simulink library "libMdl_AccIntegrator"  (R2019b)
settings: Solver=VariableStepAuto  StartTime=0.0  StopTime=10.0  RelTol=1e-3
undefined symbols (not defined in the file): DiscIntNeverNeededParam
libraries: libMdl_crossProdMat x1, libMdl_transformVect x1
settings Model: Creator=Hanno  LastModifiedBy=Hanno

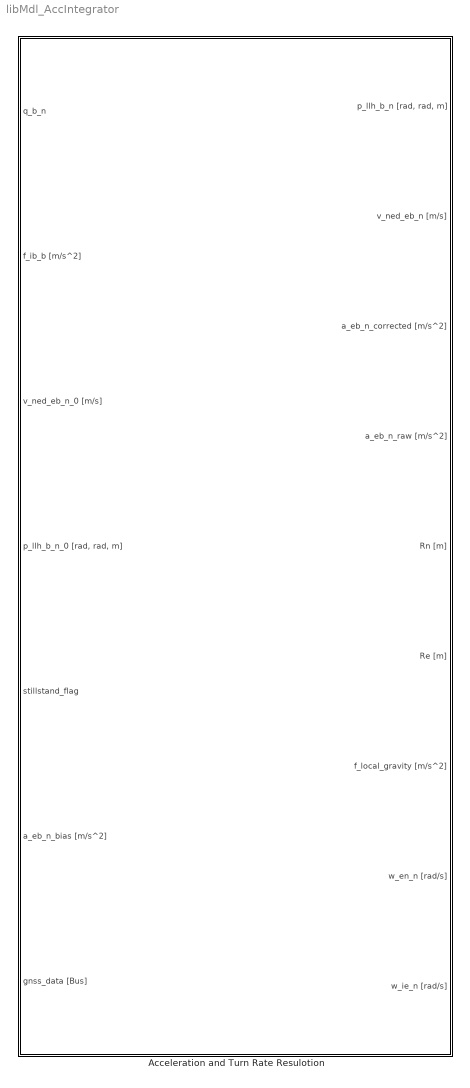
== system libMdl_AccIntegrator ==
  "Acceleration and Turn Rate Resulotion " : Subsystem  mask{mv_sample_time=-1}
      mask prompts: mv_sample_time "Sample Time:"
      mask Display:
      | str1 = sprintf('\\color{black}{\\bfINS Resolution and Integration}\n\n');
      | str2 = sprintf('Sample Time: %0.3f',mv_sample_time);
      | 
      | str = [str1,str2];
      | 
      | text( 0.5,0.5, ...
      |       str, ...
      |       'horizontalAlignment', 'center', ...
      |       'texmode','on' ...
      |     )

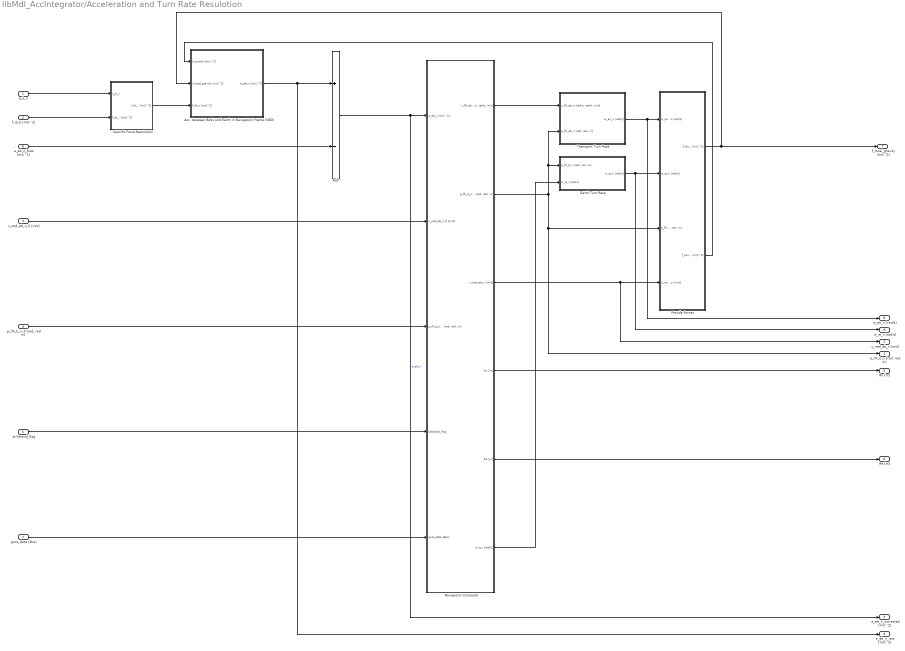
== system libMdl_AccIntegrator/Acceleration and Turn Rate Resulotion  ==
  q_b_n : Inport
  f_ib_b [m/s^2] : Inport  Port=2
  v_ned_eb_n_0 [m/s] : Inport  Port=3
  "p_llh_b_n_0 [rad, rad, m] " : Inport  Port=4
  stillstand_flag : Inport  Port=5
  a_eb_n_bias [m/s^2] : Inport  Port=6
  gnss_data [Bus] : Inport  Port=7
  Acc. between Body and Earth in Navigation Frame (NED) : Subsystem
  Add : Sum  Inputs=+-
  Earth Turn Rate : Subsystem
  Navigation Computer : Subsystem
  Pseude Forces : Subsystem
  Specific Force Resolution : Subsystem
  Transport Turn Rate : Subsystem
  "p_llh_b_n [rad, rad, m]" : Outport  VectorParamsAs1DForOutWhenUnconnected=off
  v_ned_eb_n [m/s] : Outport  Port=2  VectorParamsAs1DForOutWhenUnconnected=off
  a_eb_n_corrected [m/s^2] : Outport  Port=3  VectorParamsAs1DForOutWhenUnconnected=off
  a_eb_n_raw [m/s^2] : Outport  Port=4  VectorParamsAs1DForOutWhenUnconnected=off
  Rn [m] : Outport  Port=5  VectorParamsAs1DForOutWhenUnconnected=off
  Re [m] : Outport  Port=6  VectorParamsAs1DForOutWhenUnconnected=off
  f_local_gravity [m/s^2] : Outport  Port=7  VectorParamsAs1DForOutWhenUnconnected=off
  w_en_n [rad/s] : Outport  Port=8  VectorParamsAs1DForOutWhenUnconnected=off
  w_ie_n [rad/s] : Outport  Port=9  VectorParamsAs1DForOutWhenUnconnected=off
  wires:
  Navigation Computer/6(w_ie_i [rad/s]) -> Earth Turn Rate/2(w_ie_i [rad/s])
  a_eb_n_bias [m/s^2]/1 -> Add/2
  stillstand_flag/1 -> Navigation Computer/4(stillstand_flag)
  Add/1 -> a_eb_n_corrected [m/s^2]/1, Navigation Computer/1(a_eb_n [m/s^2])  "a_eb_n"
  Navigation Computer/5(Re [m]) -> Re [m]/1
  Navigation Computer/4(Rn [m]) -> Rn [m]/1
  Pseude Forces/1(f_local_gravity [m/s^2]) -> Acc. between Body and Earth in Navigation Frame (NED)/2(f_local_gravity [m/s^2]), f_local_gravity [m/s^2]/1
  Pseude Forces/2(f_coriolis [m/s^2]) -> Acc. between Body and Earth in Navigation Frame (NED)/1(f_coriolis [m/s^2])
  Navigation Computer/3(v_ned_eb_n [m/s]) -> Pseude Forces/4(v_ned_eb_n [m/s]), v_ned_eb_n [m/s]/1
  Earth Turn Rate/1(w_ie_n [rad/s]) -> Pseude Forces/2(w_ie_n [rad/s]), w_ie_n [rad/s]/1
  Transport Turn Rate/1(w_en_n [rad/s]) -> w_en_n [rad/s]/1, Pseude Forces/1(w_en_n [rad/s])
  Navigation Computer/1("v_llh_eb_n [rad/s, rad/s, m/s]") -> Transport Turn Rate/1("v_llh_eb_n [rad/s, rad/s, m/s]")
  Navigation Computer/2("p_llh_b_n [rad, rad, m]") -> Earth Turn Rate/1("p_llh_b_n [rad, rad, m]"), Transport Turn Rate/2("p_llh_eb_n [rad, rad, m]"), Pseude Forces/3("p_llh_eb_n [rad, rad, m]"), "p_llh_b_n [rad, rad, m]"/1
  f_ib_b [m/s^2]/1 -> Specific Force Resolution/2(f_ib_b [m/s^2])
  Specific Force Resolution/1(f_ib_n [m/s^2]) -> Acc. between Body and Earth in Navigation Frame (NED)/3(f_ib_n [m/s^2])
  "p_llh_b_n_0 [rad, rad, m] "/1 -> Navigation Computer/3("p_llh_b_n_0 [rad, rad, m]")
  Acc. between Body and Earth in Navigation Frame (NED)/1(a_eb_n [m/s^2]) -> Add/1, a_eb_n_raw [m/s^2]/1
  v_ned_eb_n_0 [m/s]/1 -> Navigation Computer/2(v_ned_eb_n_0 [m/s])
  q_b_n/1 -> Specific Force Resolution/1(q_b_n)
  gnss_data [Bus]/1 -> Navigation Computer/5(gnss_data [Bus])

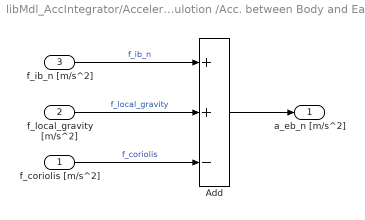
== system libMdl_AccIntegrator/Acceleration and Turn Rate Resulotion /Acc. between Body and Earth in Navigation Frame (NED) ==
  f_coriolis [m/s^2] : Inport
  f_local_gravity [m/s^2] : Inport  Port=2
  f_ib_n [m/s^2] : Inport  Port=3
  Add : Sum  Inputs=++-
  a_eb_n [m/s^2] : Outport  VectorParamsAs1DForOutWhenUnconnected=off
  wires:
  f_coriolis [m/s^2]/1 -> Add/3  "f_coriolis"
  f_local_gravity [m/s^2]/1 -> Add/2  "f_local_gravity"
  Add/1 -> a_eb_n [m/s^2]/1
  f_ib_n [m/s^2]/1 -> Add/1  "f_ib_n"

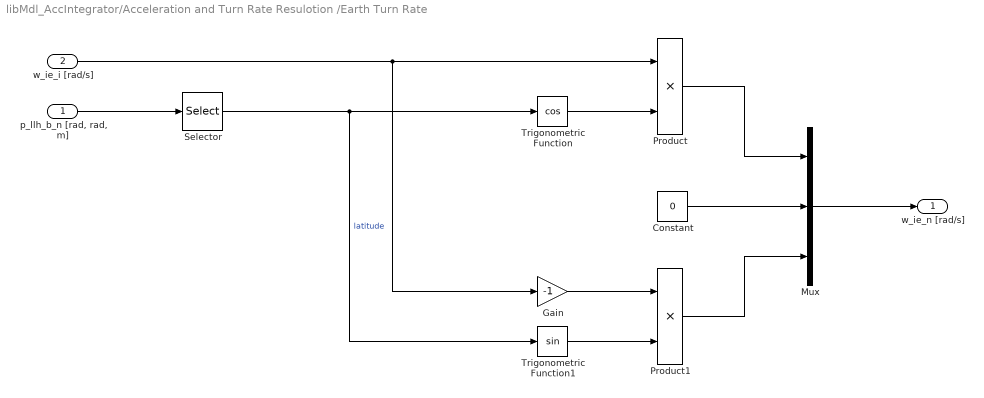
== system libMdl_AccIntegrator/Acceleration and Turn Rate Resulotion /Earth Turn Rate ==
  "p_llh_b_n [rad, rad, m]" : Inport
  w_ie_i [rad/s] : Inport  Port=2
  Constant : Constant  Value=0
  Gain : Gain  Gain=-1
  Mux : Mux  Inputs=3
  Product : Product
  Product1 : Product
  Selector : Selector  InputPortWidth=3  IndexOptions=Index vector (dialog)  Indices=1  OutputSizes=1
  Trigonometric Function : Trigonometry  Operator=cos
  Trigonometric Function1 : Trigonometry
  w_ie_n [rad/s] : Outport  VectorParamsAs1DForOutWhenUnconnected=off
  wires:
  Product1/1 -> Mux/3
  Product/1 -> Mux/1
  Constant/1 -> Mux/2
  Gain/1 -> Product1/1
  Mux/1 -> w_ie_n [rad/s]/1
  Trigonometric Function1/1 -> Product1/2
  Trigonometric Function/1 -> Product/2
  w_ie_i [rad/s]/1 -> Product/1, Gain/1
  Selector/1 -> Trigonometric Function/1, Trigonometric Function1/1  "latitude"
  "p_llh_b_n [rad, rad, m]"/1 -> Selector/1

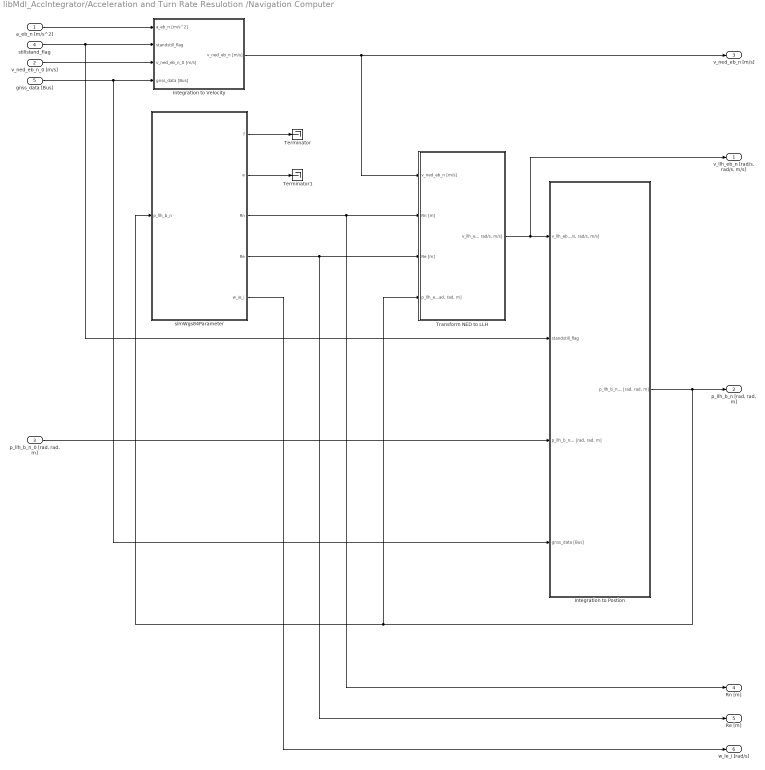
== system libMdl_AccIntegrator/Acceleration and Turn Rate Resulotion /Navigation Computer ==
  a_eb_n [m/s^2] : Inport
  v_ned_eb_n_0 [m/s] : Inport  Port=2
  "p_llh_b_n_0 [rad, rad, m]" : Inport  Port=3
  stillstand_flag : Inport  Port=4
  gnss_data [Bus] : Inport  Port=5
  Integration to Postion : Subsystem
  Integration to Velocity : Subsystem
  Terminator : Terminator
  Terminator1 : Terminator
  Transform NED to LLH : Subsystem
  simWgs84Parameter : MATLAB Function  TreatAsAtomicUnit=on  SystemSampleTime=mv_sample_time  mask{mv_sample_time=-1}
      mask prompts: mv_sample_time "Sample Time:"
  "v_llh_eb_n [rad/s, rad/s, m/s]" : Outport  VectorParamsAs1DForOutWhenUnconnected=off
  "p_llh_b_n [rad, rad, m]" : Outport  Port=2  VectorParamsAs1DForOutWhenUnconnected=off
  v_ned_eb_n [m/s] : Outport  Port=3  VectorParamsAs1DForOutWhenUnconnected=off
  Rn [m] : Outport  Port=4  VectorParamsAs1DForOutWhenUnconnected=off
  Re [m] : Outport  Port=5  VectorParamsAs1DForOutWhenUnconnected=off
  w_ie_i [rad/s] : Outport  Port=6  VectorParamsAs1DForOutWhenUnconnected=off
  wires:
  simWgs84Parameter/5(w_ie_i) -> w_ie_i [rad/s]/1
  stillstand_flag/1 -> Integration to Postion/2(standstill_flag), Integration to Velocity/2(standstill_flag)
  simWgs84Parameter/2(e) -> Terminator1/1
  simWgs84Parameter/1(f) -> Terminator/1
  simWgs84Parameter/4(Re) -> Transform NED to LLH/3(Re [m]), Re [m]/1
  simWgs84Parameter/3(Rn) -> Transform NED to LLH/2(Rn [m]), Rn [m]/1
  Integration to Postion/1("p_llh_b_n [rad, rad, m]") -> "p_llh_b_n [rad, rad, m]"/1, Transform NED to LLH/4("p_llh_eb_n [rad, rad, m]"), simWgs84Parameter/1(p_llh_b_n)
  "p_llh_b_n_0 [rad, rad, m]"/1 -> Integration to Postion/3("p_llh_b_n_0 [rad, rad, m]")
  v_ned_eb_n_0 [m/s]/1 -> Integration to Velocity/3(v_ned_eb_n_0 [m/s])
  Integration to Velocity/1(v_ned_eb_n [m/s]) -> Transform NED to LLH/1(v_ned_eb_n [m/s]), v_ned_eb_n [m/s]/1
  a_eb_n [m/s^2]/1 -> Integration to Velocity/1(a_eb_n [m/s^2])
  Transform NED to LLH/1("v_llh_eb_n [rad/s, rad/s, m/s]") -> "v_llh_eb_n [rad/s, rad/s, m/s]"/1, Integration to Postion/1("v_llh_eb_n [rad/s, rad/s, m/s]")
  gnss_data [Bus]/1 -> Integration to Velocity/4(gnss_data [Bus]), Integration to Postion/4(gnss_data [Bus])

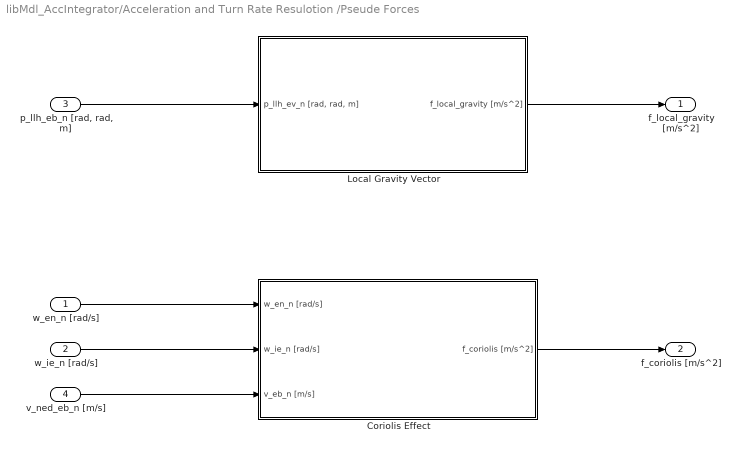
== system libMdl_AccIntegrator/Acceleration and Turn Rate Resulotion /Pseude Forces ==
  w_en_n [rad/s] : Inport
  w_ie_n [rad/s] : Inport  Port=2
  "p_llh_eb_n [rad, rad, m]" : Inport  Port=3
  v_ned_eb_n [m/s] : Inport  Port=4
  Coriolis Effect : Subsystem
  Local Gravity Vector : Subsystem
      settings: AttributesFormatString="Local Gravity Model according to: D. Titterton and J. Westen, \"Strapdown Inertial Navigation Technology\", p. 57, IET, 2004"
  f_local_gravity [m/s^2] : Outport  VectorParamsAs1DForOutWhenUnconnected=off
  f_coriolis [m/s^2] : Outport  Port=2  VectorParamsAs1DForOutWhenUnconnected=off
  wires:
  Coriolis Effect/1(f_coriolis [m/s^2]) -> f_coriolis [m/s^2]/1
  Local Gravity Vector/1(f_local_gravity [m/s^2]) -> f_local_gravity [m/s^2]/1
  v_ned_eb_n [m/s]/1 -> Coriolis Effect/3(v_eb_n [m/s])
  "p_llh_eb_n [rad, rad, m]"/1 -> Local Gravity Vector/1("p_llh_ev_n [rad, rad, m]")
  w_ie_n [rad/s]/1 -> Coriolis Effect/2(w_ie_n [rad/s])
  w_en_n [rad/s]/1 -> Coriolis Effect/1(w_en_n [rad/s])

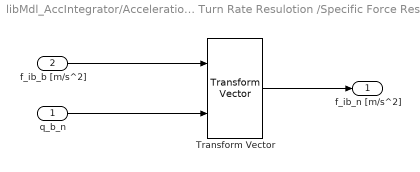
== system libMdl_AccIntegrator/Acceleration and Turn Rate Resulotion /Specific Force Resolution ==
  q_b_n : Inport
  f_ib_b [m/s^2] : Inport  Port=2
  Transform Vector : libMdl_transformVect/Transform Vector  SystemSampleTime=-1  Latency=0  AutoFrameSizeCalculation=off
  f_ib_n [m/s^2] : Outport  VectorParamsAs1DForOutWhenUnconnected=off
  wires:
  f_ib_b [m/s^2]/1 -> Transform Vector/1
  Transform Vector/1 -> f_ib_n [m/s^2]/1
  q_b_n/1 -> Transform Vector/2

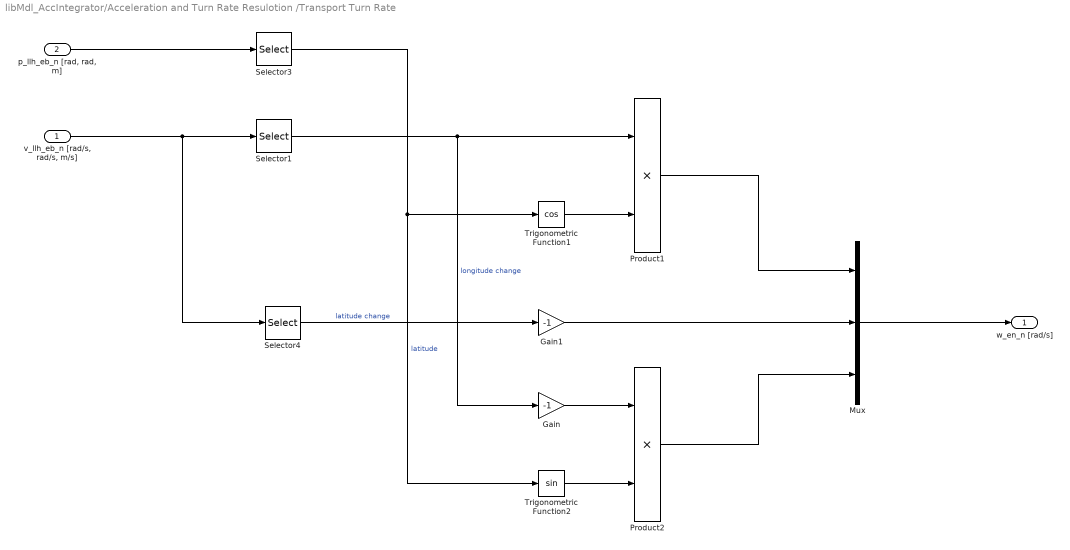
== system libMdl_AccIntegrator/Acceleration and Turn Rate Resulotion /Transport Turn Rate ==
  "v_llh_eb_n [rad/s, rad/s, m/s]" : Inport
  "p_llh_eb_n [rad, rad, m]" : Inport  Port=2
  Gain : Gain  Gain=-1
  Gain1 : Gain  Gain=-1
  Mux : Mux  Inputs=3
  Product1 : Product
  Product2 : Product
  Selector1 : Selector  InputPortWidth=3  IndexOptions=Index vector (dialog)  Indices=2  OutputSizes=1
  Selector3 : Selector  InputPortWidth=3  IndexOptions=Index vector (dialog)  Indices=1  OutputSizes=1
  Selector4 : Selector  InputPortWidth=3  IndexOptions=Index vector (dialog)  Indices=1  OutputSizes=1
  Trigonometric Function1 : Trigonometry  Operator=cos
  Trigonometric Function2 : Trigonometry
  w_en_n [rad/s] : Outport  VectorParamsAs1DForOutWhenUnconnected=off
  wires:
  Product2/1 -> Mux/3
  Product1/1 -> Mux/1
  Gain1/1 -> Mux/2
  Gain/1 -> Product2/1
  Trigonometric Function2/1 -> Product2/2
  Selector4/1 -> Gain1/1  "latitude change"
  Selector1/1 -> Product1/1, Gain/1  "longitude change"
  Selector3/1 -> Trigonometric Function1/1, Trigonometric Function2/1  "latitude"
  Trigonometric Function1/1 -> Product1/2
  Mux/1 -> w_en_n [rad/s]/1
  "p_llh_eb_n [rad, rad, m]"/1 -> Selector3/1
  "v_llh_eb_n [rad/s, rad/s, m/s]"/1 -> Selector1/1, Selector4/1

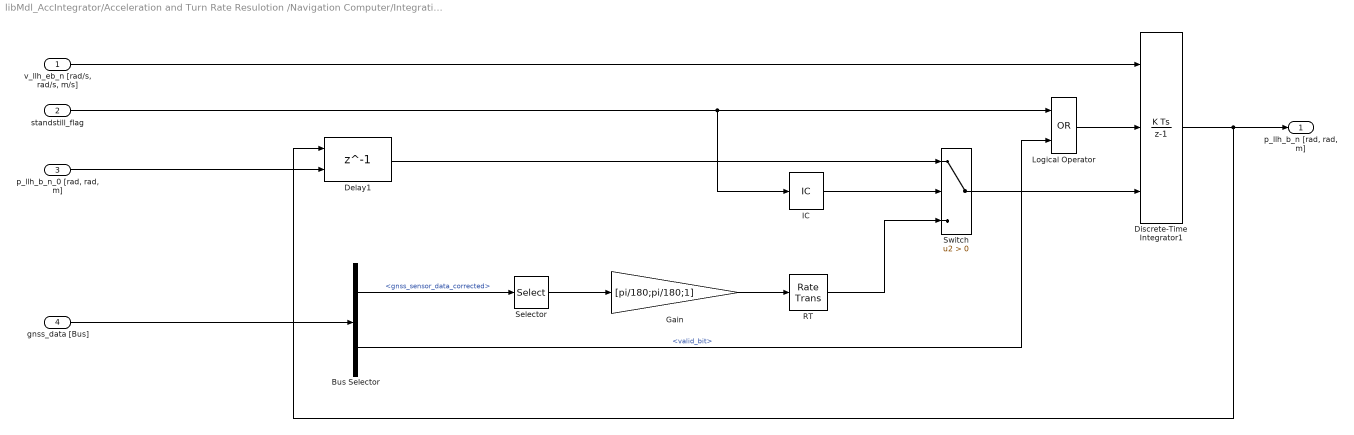
== system libMdl_AccIntegrator/Acceleration and Turn Rate Resulotion /Navigation Computer/Integration to Postion ==
  "v_llh_eb_n [rad/s, rad/s, m/s]" : Inport
  standstill_flag : Inport  Port=2
  "p_llh_b_n_0 [rad, rad, m]" : Inport  Port=3
  gnss_data [Bus] : Inport  Port=4
  Bus Selector : BusSelector  OutputSignals=gnss_sensor_data_corrected,valid_bit
  Delay1 : Delay  DelayLength=1  InitialConditionSource=Input port
      settings: InputPortMap=u0,p4
  Discrete-Time Integrator1 : DiscreteIntegrator  ExternalReset=sampled level  InitialConditionSource=external  SampleTime=mv_sample_time  ICPrevOutput=DiscIntNeverNeededParam  ICPrevScaledInput=DiscIntNeverNeededParam
  Gain : Gain  Gain=[pi/180;pi/180;1]
  IC : InitialCondition
  Logical Operator : Logic  Operator=OR  AllPortsSameDT=off  OutDataTypeStr=boolean
  RT : RateTransition
  Selector : Selector  InputPortWidth=7  IndexOptions=Index vector (dialog)  Indices=1:3  OutputSizes=1
  Switch : Switch  Criteria=u2 > Threshold
  "p_llh_b_n [rad, rad, m]" : Outport
  wires:
  Selector/1 -> Gain/1
  RT/1 -> Switch/3
  Bus Selector/2 -> Logical Operator/2  "<valid_bit>"
  Logical Operator/1 -> Discrete-Time Integrator1/2
  Delay1/1 -> Switch/1
  Switch/1 -> Discrete-Time Integrator1/3
  "v_llh_eb_n [rad/s, rad/s, m/s]"/1 -> Discrete-Time Integrator1/1
  gnss_data [Bus]/1 -> Bus Selector/1
  Discrete-Time Integrator1/1 -> "p_llh_b_n [rad, rad, m]"/1, Delay1/1
  Bus Selector/1 -> Selector/1  "<gnss_sensor_data_corrected>"
  standstill_flag/1 -> Logical Operator/1, IC/1
  "p_llh_b_n_0 [rad, rad, m]"/1 -> Delay1/2
  Gain/1 -> RT/1
  IC/1 -> Switch/2

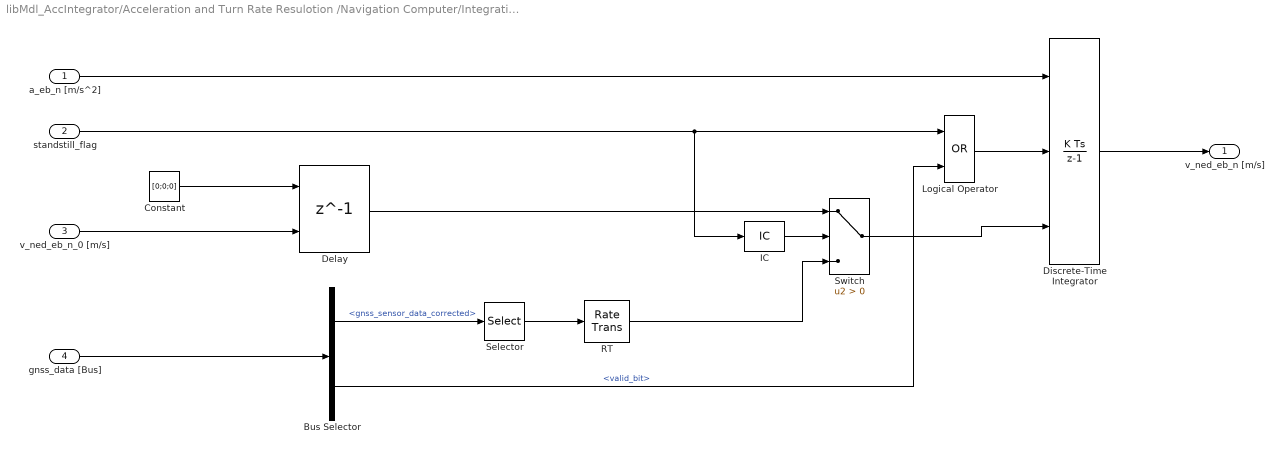
== system libMdl_AccIntegrator/Acceleration and Turn Rate Resulotion /Navigation Computer/Integration to Velocity ==
  a_eb_n [m/s^2] : Inport
  standstill_flag : Inport  Port=2
  v_ned_eb_n_0 [m/s] : Inport  Port=3
  gnss_data [Bus] : Inport  Port=4
  Bus Selector : BusSelector  OutputSignals=gnss_sensor_data_corrected,valid_bit
  Constant : Constant  Value=[0;0;0]
  Delay : Delay  DelayLength=1  InitialConditionSource=Input port
      settings: InputPortMap=u0,p4
  Discrete-Time Integrator : DiscreteIntegrator  ExternalReset=sampled level  InitialConditionSource=external  SampleTime=mv_sample_time  ICPrevOutput=DiscIntNeverNeededParam  ICPrevScaledInput=DiscIntNeverNeededParam
  IC : InitialCondition
  Logical Operator : Logic  Operator=OR  AllPortsSameDT=off  OutDataTypeStr=boolean
  RT : RateTransition
  Selector : Selector  InputPortWidth=7  IndexOptions=Index vector (dialog)  Indices=4:6  OutputSizes=1
  Switch : Switch  Criteria=u2 > Threshold
  v_ned_eb_n [m/s] : Outport
  wires:
  a_eb_n [m/s^2]/1 -> Discrete-Time Integrator/1
  Discrete-Time Integrator/1 -> v_ned_eb_n [m/s]/1
  v_ned_eb_n_0 [m/s]/1 -> Delay/2
  Logical Operator/1 -> Discrete-Time Integrator/2
  Constant/1 -> Delay/1
  Bus Selector/1 -> Selector/1  "<gnss_sensor_data_corrected>"
  Bus Selector/2 -> Logical Operator/2  "<valid_bit>"
  gnss_data [Bus]/1 -> Bus Selector/1
  Switch/1 -> Discrete-Time Integrator/3
  standstill_flag/1 -> Logical Operator/1, IC/1
  Delay/1 -> Switch/1
  Selector/1 -> RT/1
  RT/1 -> Switch/3
  IC/1 -> Switch/2

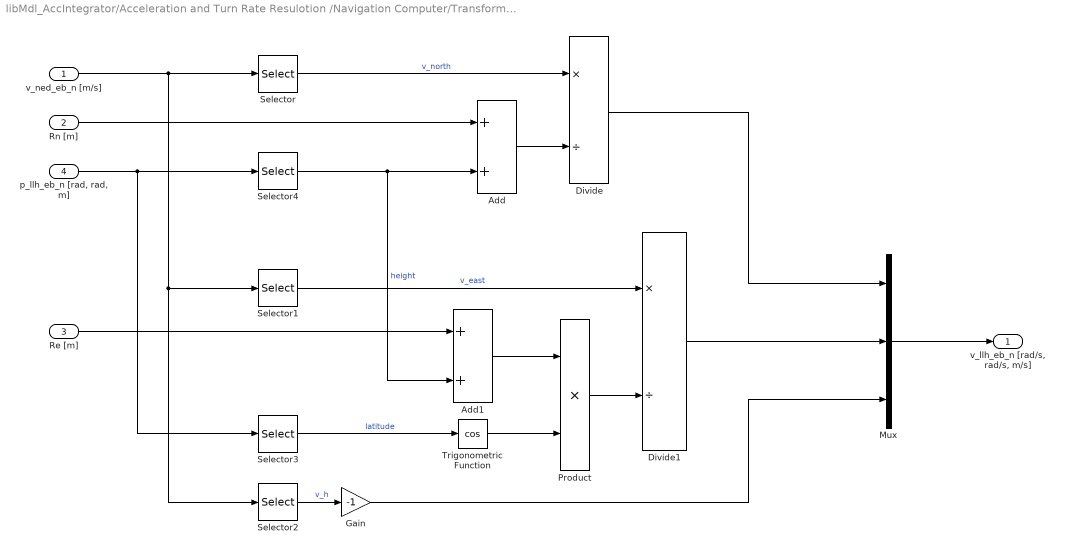
== system libMdl_AccIntegrator/Acceleration and Turn Rate Resulotion /Navigation Computer/Transform NED to LLH ==
  v_ned_eb_n [m/s] : Inport
  Rn [m] : Inport  Port=2
  Re [m] : Inport  Port=3
  "p_llh_eb_n [rad, rad, m]" : Inport  Port=4
  Add : Sum
  Add1 : Sum
  Divide : Product  Inputs=*/
  Divide1 : Product  Inputs=*/
  Gain : Gain  Gain=-1
  Mux : Mux  Inputs=3
  Product : Product
  Selector : Selector  InputPortWidth=3  IndexOptions=Index vector (dialog)  Indices=1  OutputSizes=1
  Selector1 : Selector  InputPortWidth=3  IndexOptions=Index vector (dialog)  Indices=2  OutputSizes=1
  Selector2 : Selector  InputPortWidth=3  IndexOptions=Index vector (dialog)  Indices=3  OutputSizes=1
  Selector3 : Selector  InputPortWidth=3  IndexOptions=Index vector (dialog)  Indices=1  OutputSizes=1
  Selector4 : Selector  InputPortWidth=3  IndexOptions=Index vector (dialog)  Indices=3  OutputSizes=1
  Trigonometric Function : Trigonometry  Operator=cos
  "v_llh_eb_n [rad/s, rad/s, m/s]" : Outport  VectorParamsAs1DForOutWhenUnconnected=off
  wires:
  "p_llh_eb_n [rad, rad, m]"/1 -> Selector4/1, Selector3/1
  Trigonometric Function/1 -> Product/2
  Selector3/1 -> Trigonometric Function/1  "latitude"
  Product/1 -> Divide1/2
  Mux/1 -> "v_llh_eb_n [rad/s, rad/s, m/s]"/1
  Gain/1 -> Mux/3
  Divide/1 -> Mux/1
  Divide1/1 -> Mux/2
  Re [m]/1 -> Add1/1
  Selector4/1 -> Add/2, Add1/2  "height"
  Rn [m]/1 -> Add/1
  Add1/1 -> Product/1
  Add/1 -> Divide/2
  Selector1/1 -> Divide1/1  "v_east"
  Selector/1 -> Divide/1  "v_north"
  Selector2/1 -> Gain/1  "v_h"
  v_ned_eb_n [m/s]/1 -> Selector/1, Selector1/1, Selector2/1

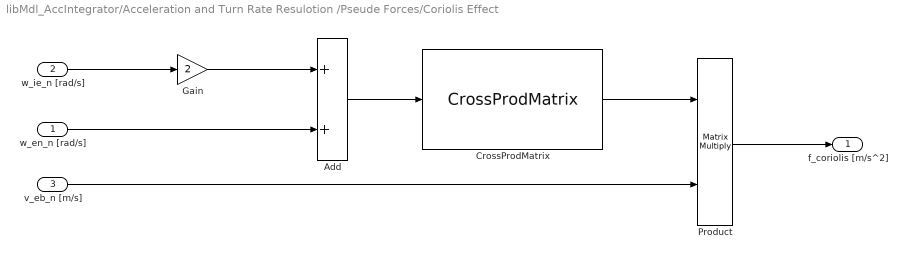
== system libMdl_AccIntegrator/Acceleration and Turn Rate Resulotion /Pseude Forces/Coriolis Effect ==
  w_en_n [rad/s] : Inport
  w_ie_n [rad/s] : Inport  Port=2
  v_eb_n [m/s] : Inport  Port=3
  Add : Sum
  CrossProdMatrix : libMdl_crossProdMat/CrossProdMatrix  SystemSampleTime=-1  Latency=0  AutoFrameSizeCalculation=off
  Gain : Gain  Gain=2
  Product : Product  Multiplication=Matrix(*)
  f_coriolis [m/s^2] : Outport  VectorParamsAs1DForOutWhenUnconnected=off
  wires:
  Product/1 -> f_coriolis [m/s^2]/1
  v_eb_n [m/s]/1 -> Product/2
  CrossProdMatrix/1 -> Product/1
  Add/1 -> CrossProdMatrix/1
  w_en_n [rad/s]/1 -> Add/2
  Gain/1 -> Add/1
  w_ie_n [rad/s]/1 -> Gain/1

== system libMdl_AccIntegrator/Acceleration and Turn Rate Resulotion /Pseude Forces/Local Gravity Vector ==
  "p_llh_ev_n [rad, rad, m]" : Inport
  simLocalGravityModel : MATLAB Function  TreatAsAtomicUnit=on
  f_local_gravity [m/s^2] : Outport  VectorParamsAs1DForOutWhenUnconnected=off
  wires:
  simLocalGravityModel/1(f_local_gravity) -> f_local_gravity [m/s^2]/1
  "p_llh_ev_n [rad, rad, m]"/1 -> simLocalGravityModel/1(p_llh_ev_nu)

== matlab function libMdl_AccIntegrator/Acceleration and Turn Rate Resulotion /Pseude Forces/Local Gravity Vector/simLocalGravityModel ==
  data: p_llh_ev_nu input; f_local_gravity output
function f_local_gravity = simLocalGravityModel(p_llh_ev_nu)

g0 = 9.780318;
g1 = 5.3024e-3;
g2 = 5.9e-6;

dgdh0 = 3.0877e-6;
dgdh1 = 1.39e-3;

L = p_llh_ev_nu(1);
h = p_llh_ev_nu(3);

g_sealevel = g0*(1+g1*sin(L)^2-g2*sin(2*L)^2);
dgdh = -dgdh0*(1-dgdh1*sin(L)^2);

local_gravity = g_sealevel + dgdh*h;

f_local_gravity = [0;0;local_gravity];

end % function

== matlab function libMdl_AccIntegrator/Acceleration and Turn Rate Resulotion /Navigation Computer/simWgs84Parameter ==
  settings: updateMethod=DISCRETE  sampleTime=mv_sample_time
  data: p_llh_b_n input; f output; e output; Rn output; Re output; w_ie_i output
function [f,e,Rn,Re,w_ie_i] = simWgs84Parameter(p_llh_b_n)

[f,e,Rn,Re,w_ie_i] = getWgs84Parameter(p_llh_b_n);

end % function
